simulink model "DieuKhienPhanHoiTrangThaiGanDiemCuc2222"  (R2014a)
settings: Solver=ode45  StartTime=0.0  StopTime=15  RelTol=1e-3
settings Model: Creator=tri  LastModifiedBy=tri

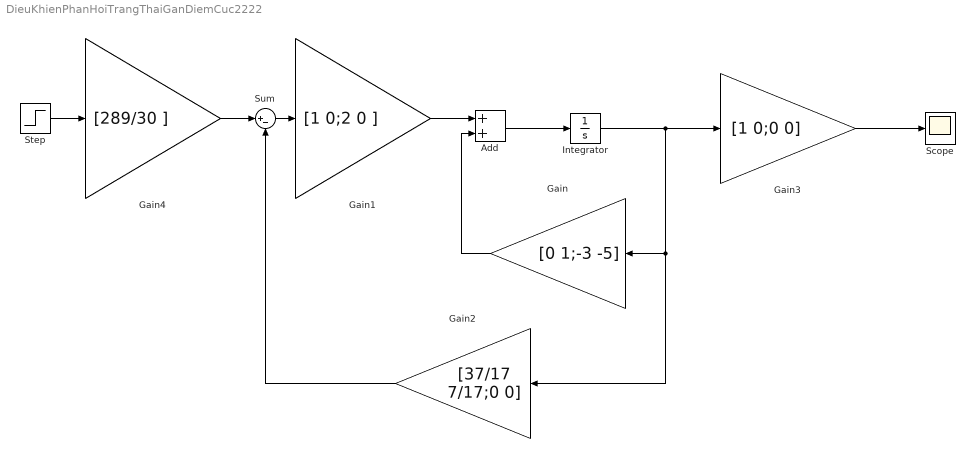
== system DieuKhienPhanHoiTrangThaiGanDiemCuc2222 ==
  Add : Sum
  Gain : Gain  Gain=[0 1;-3 -5]
  Gain1 : Gain  Gain=[1 0;2 0 ]
  Gain2 : Gain  Gain=[37/17 7/17;0 0]
  Gain3 : Gain  Gain=[1 0;0 0]
  Gain4 : Gain  Gain=[289/30 ]
  Integrator : Integrator
  Scope : Scope
  Step : Step  After=10  SampleTime=0
  Sum : Sum  Inputs=|+-
  wires:
  Gain/1 -> Add/2
  Add/1 -> Integrator/1
  Integrator/1 -> Gain3/1, Gain2/1, Gain/1
  Gain1/1 -> Add/1
  Gain3/1 -> Scope/1
  Gain2/1 -> Sum/2
  Sum/1 -> Gain1/1
  Step/1 -> Gain4/1
  Gain4/1 -> Sum/1
